simulink model "L0401"  (R2022b)
settings: Solver=ode5  StartTime=0.0  StopTime=100.0  FixedStep=0.001  RelTol=1e-3
values from neighbouring files (symbols this model uses):
  c = double(c)    [vehicle.m]
  hend = 22.55    [vehicle.m]
  hstart = 22.5    [vehicle.m]
  k = double(k)    [vehicle.m]
  m = 1000    [vehicle.m]
settings Model: Creator=Andrey  LastModifiedBy=Andrey

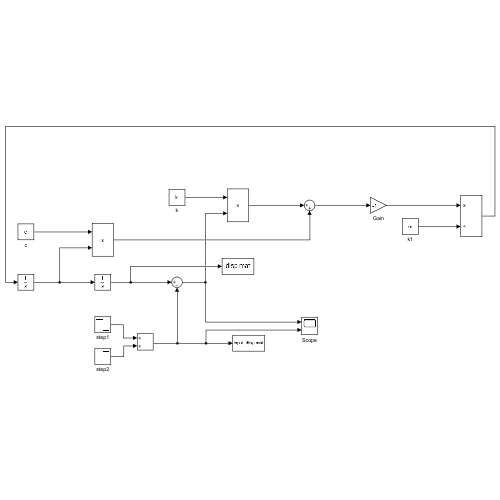
[thumbnail: Simulink's stored preview of the top-level diagram]
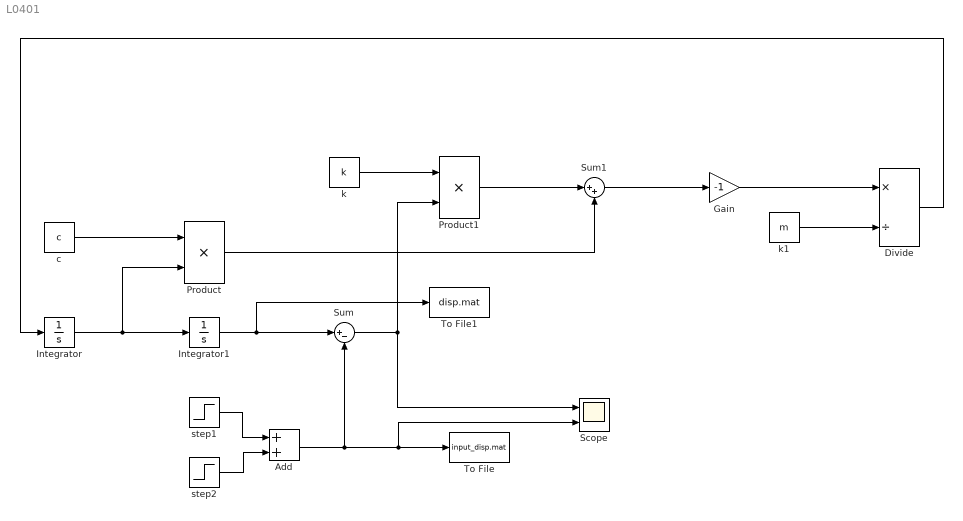
== system L0401 ==
  Add : Sum
  Divide : Product  Inputs=*/
  Gain : Gain  Gain=-1
  Integrator : Integrator
  Integrator1 : Integrator
  Product : Product
  Product1 : Product
  Scope : Scope  NumInputPorts=2
  Sum : Sum  Inputs=|+-
  Sum1 : Sum  Inputs=|++
  To File : ToFile  Filename=input_disp.mat  MatrixName=input_disp  SaveFormat=Timeseries
  To File1 : ToFile  Filename=disp.mat  MatrixName=disp  SaveFormat=Timeseries
  c : Constant  Value=c
  k : Constant  Value=k
  k1 : Constant  Value=m
  step1 : Step  Time=hstart  After=-0.15  SampleTime=0
  step2 : Step  Time=hend  After=0.15  SampleTime=0
  wires:
  Integrator/1 -> Product/2, Integrator1/1
  c/1 -> Product/1
  Integrator1/1 -> To File1/1, Sum/1
  Sum/1 -> Product1/2, Scope/1
  k/1 -> Product1/1
  Product1/1 -> Sum1/1
  Product/1 -> Sum1/2
  Sum1/1 -> Gain/1
  Gain/1 -> Divide/1
  k1/1 -> Divide/2
  Divide/1 -> Integrator/1
  step1/1 -> Add/1
  Add/1 -> Sum/2, Scope/2, To File/1
  step2/1 -> Add/2
